simulink model "hexacop"  (R2017a)
settings: Solver=VariableStepAuto  StartTime=0.0  StopTime=10.0  RelTol=1e-3
values from neighbouring files (symbols this model uses):
  b = 3.13*exp(-5)    [Hexacopter_values.m]    (also in values.m)
  d = 7.5*exp(-7)    [values.m]
  g = 9.81    [values.m]
  Jr = 6*exp(-5)    [Hexacopter_values.m]    (also in values.m)
  Jxx = 7.5*10^-3    (= 0.0075)    [Hexacopter_values.m]    (also in values.m = 7.5*exp(-3))
  Jyy = 7.5*10^-3    (= 0.0075)    [Hexacopter_values.m]    (also in values.m = 7.5*exp(-3))
  Jzz = 1.3*10^-2    (= 0.013)    [Hexacopter_values.m]    (also in values.m = 1.3*exp(-2))
  Kfax = 0.1    [Hexacopter_values.m]    (also in values.m)
  Kfay = 0.1    [Hexacopter_values.m]    (also in values.m)
  Kfaz = 0.15    [Hexacopter_values.m]    (also in values.m)
  kftx = 1.5    [values.m]
  kfty = 0.1    [values.m]
  kftz = 1.9    [values.m]
  l = 0.23    [Hexacopter_values.m]    (also in values.m = 1)
  m = 0.65    [Hexacopter_values.m]    (also in values.m = 5)
libraries: simulink x4
settings Model: Creator=Pari  LastModifiedBy=Jash

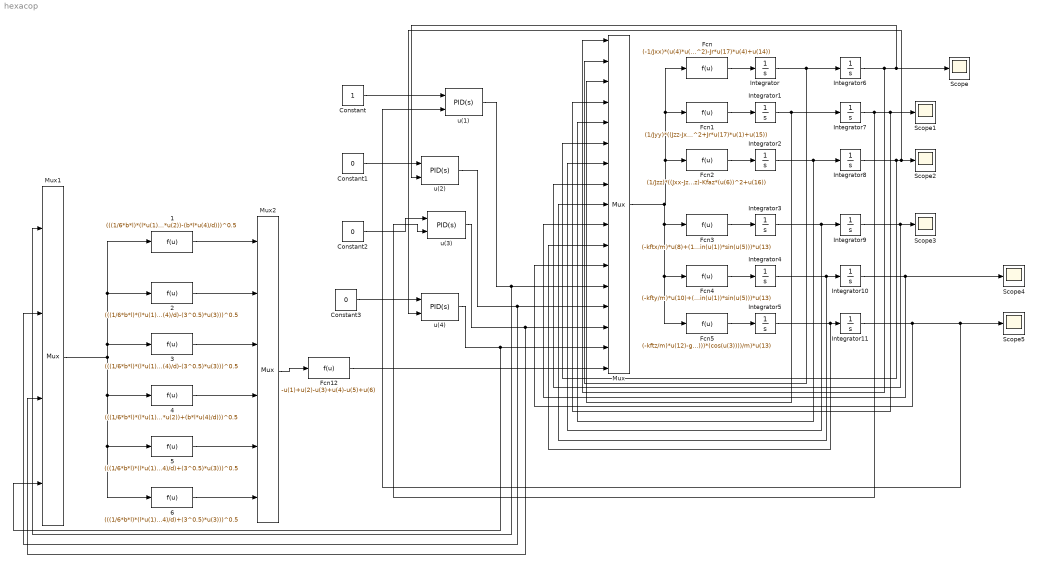
== system hexacop ==
  1 : Fcn  Expr=(((1/6*b*l)*(l*u(1)+2*u(2))-(b*l*u(4)/d)))^0.5
  2 : Fcn  Expr=(((1/6*b*l)*(l*u(1)+u(2))+(b*l*u(4)/d)-(3^0.5)*u(3)))^0.5
  3 : Fcn  Expr=(((1/6*b*l)*(l*u(1)-u(2))-(b*l*u(4)/d)-(3^0.5)*u(3)))^0.5
  4 : Fcn  Expr=(((1/6*b*l)*(l*u(1)-2*u(2))+(b*l*u(4)/d)))^0.5
  5 : Fcn  Expr=(((1/6*b*l)*(l*u(1)-u(2))-(b*l*u(4)/d)+(3^0.5)*u(3)))^0.5
  6 : Fcn  Expr=(((1/6*b*l)*(l*u(1)+u(2))+(b*l*u(4)/d)+(3^0.5)*u(3)))^0.5
  Constant : Constant
  Constant1 : Constant  Value=0
  Constant2 : Constant  Value=0
  Constant3 : Constant  Value=0
  Fcn : Fcn  Expr=(-1/Jxx)*(u(4)*u(6)*(Jyy-Jzz)*Kfax*((u(2))^2)-Jr*u(17)*u(4)+u(14))
  Fcn1 : Fcn  Expr=(1/Jyy)*((Jzz-Jxx)-Kfay*(u(3))^2+Jr*u(17)*u(1)+u(15))
  Fcn12 : Fcn  Expr=-u(1)+u(2)-u(3)+u(4)-u(5)+u(6)
  Fcn2 : Fcn  Expr=(1/Jzz)*((Jxx-Jzz)-Kfaz*(u(6))^2+u(16))
  Fcn3 : Fcn  Expr=(-kftx/m)*u(8)+(1/m)*((cos(u(1))*cos(u(5))*sin(u(3)))+sin(u(1))*sin(u(5)))*u(13)
  Fcn4 : Fcn  Expr=(-kfty/m)*u(10)+(1/m)*((cos(u(1))*sin(u(3))*sin(u(5)))-sin(u(1))*sin(u(5)))*u(13)
  Fcn5 : Fcn  Expr=(-kftz/m)*u(12)-g+(((cos(u(1)))*(cos(u(3))))/m)*u(13)
  Integrator{,1..11} (12 alike) : Integrator
  Mux : Mux  Inputs=17
  Mux1 : Mux
  Mux2 : Mux  Inputs=6
  Scope{,1..5} (6 alike) : Scope
  u(1) : simulink/Continuous/PID Controller (2DOF)  Controller=PID  TimeDomain=Continuous-time  SampleTime=-1  IntegratorMethod=Forward Euler  FilterMethod=Forward Euler  Form=Parallel  UseFilter=on  ControllerParametersSource=internal  P=26.2943879402193  I=7.16633798011478  D=21.031507768883  N=46.9240700820104  b=0.842025544995177  c=0.00338936172316472  InitialConditionSource=internal  InitialConditionForIntegrator=0  InitialConditionForFilter=0  ExternalReset=none  LimitOutput=off  UpperSaturationLimit=inf  LowerSaturationLimit=-inf  LinearizeAsGain=on  AntiWindupMode=none  Kb=1  TrackingMode=off  Kt=1  PParamMin=[]  PParamMax=[]  IParamMin=[]  IParamMax=[]  DParamMin=[]  DParamMax=[]  NParamMin=[]  NParamMax=[]  bParamMin=[]  bParamMax=[]  cParamMin=[]  cParamMax=[]  KbParamMin=[]  KbParamMax=[]  KtParamMin=[]  KtParamMax=[]  POutMin=[]  POutMax=[]  IOutMin=[]  IOutMax=[]  DOutMin=[]  DOutMax=[]  NOutMin=[]  NOutMax=[]  bOutMin=[]  bOutMax=[]  cOutMin=[]  cOutMax=[]  KbOutMin=[]  KbOutMax=[]  KtOutMin=[]  KtOutMax=[]  IntegratorOutMin=[]  IntegratorOutMax=[]  FilterOutMin=[]  FilterOutMax=[]  SumOutMin=[]  SumOutMax=[]  Sum1OutMin=[]  Sum1OutMax=[]  Sum2OutMin=[]  Sum2OutMax=[]  Sum3OutMin=[]  Sum3OutMax=[]  SumI1OutMin=[]  SumI1OutMax=[]  SumI2OutMin=[]  SumI2OutMax=[]  SumI3OutMin=[]  SumI3OutMax=[]  SumDOutMin=[]  SumDOutMax=[]  SaturationOutMin=[]  SaturationOutMax=[]  IntegratorContinuousStateAttributes=''  IntegratorStateMustResolveToSignalObject=off  IntegratorRTWStateStorageClass=Auto  FilterContinuousStateAttributes=''  FilterStateMustResolveToSignalObject=off  FilterRTWStateStorageClass=Auto  DifferentiatorICPrevScaledInput=0  DifferentiatorOutMin=[]  DifferentiatorOutMax=[]  InitialConditionSetting=State (most efficient)
  u(2) : simulink/Continuous/PID Controller (2DOF)  Controller=PID  TimeDomain=Continuous-time  SampleTime=-1  IntegratorMethod=Forward Euler  FilterMethod=Forward Euler  Form=Parallel  UseFilter=on  ControllerParametersSource=internal  P=1  I=1  D=0  N=100  b=1  c=1  InitialConditionSource=internal  InitialConditionForIntegrator=0  InitialConditionForFilter=0  ExternalReset=none  LimitOutput=off  UpperSaturationLimit=inf  LowerSaturationLimit=-inf  LinearizeAsGain=on  AntiWindupMode=none  Kb=1  TrackingMode=off  Kt=1  PParamMin=[]  PParamMax=[]  IParamMin=[]  IParamMax=[]  DParamMin=[]  DParamMax=[]  NParamMin=[]  NParamMax=[]  bParamMin=[]  bParamMax=[]  cParamMin=[]  cParamMax=[]  KbParamMin=[]  KbParamMax=[]  KtParamMin=[]  KtParamMax=[]  POutMin=[]  POutMax=[]  IOutMin=[]  IOutMax=[]  DOutMin=[]  DOutMax=[]  NOutMin=[]  NOutMax=[]  bOutMin=[]  bOutMax=[]  cOutMin=[]  cOutMax=[]  KbOutMin=[]  KbOutMax=[]  KtOutMin=[]  KtOutMax=[]  IntegratorOutMin=[]  IntegratorOutMax=[]  FilterOutMin=[]  FilterOutMax=[]  SumOutMin=[]  SumOutMax=[]  Sum1OutMin=[]  Sum1OutMax=[]  Sum2OutMin=[]  Sum2OutMax=[]  Sum3OutMin=[]  Sum3OutMax=[]  SumI1OutMin=[]  SumI1OutMax=[]  SumI2OutMin=[]  SumI2OutMax=[]  SumI3OutMin=[]  SumI3OutMax=[]  SumDOutMin=[]  SumDOutMax=[]  SaturationOutMin=[]  SaturationOutMax=[]  IntegratorContinuousStateAttributes=''  IntegratorStateMustResolveToSignalObject=off  IntegratorRTWStateStorageClass=Auto  FilterContinuousStateAttributes=''  FilterStateMustResolveToSignalObject=off  FilterRTWStateStorageClass=Auto  DifferentiatorICPrevScaledInput=0  DifferentiatorOutMin=[]  DifferentiatorOutMax=[]  InitialConditionSetting=State (most efficient)
  u(3) : simulink/Continuous/PID Controller (2DOF)  Controller=PID  TimeDomain=Continuous-time  SampleTime=-1  IntegratorMethod=Forward Euler  FilterMethod=Forward Euler  Form=Parallel  UseFilter=on  ControllerParametersSource=internal  P=1  I=1  D=0  N=100  b=1  c=1  InitialConditionSource=internal  InitialConditionForIntegrator=0  InitialConditionForFilter=0  ExternalReset=none  LimitOutput=off  UpperSaturationLimit=inf  LowerSaturationLimit=-inf  LinearizeAsGain=on  AntiWindupMode=none  Kb=1  TrackingMode=off  Kt=1  PParamMin=[]  PParamMax=[]  IParamMin=[]  IParamMax=[]  DParamMin=[]  DParamMax=[]  NParamMin=[]  NParamMax=[]  bParamMin=[]  bParamMax=[]  cParamMin=[]  cParamMax=[]  KbParamMin=[]  KbParamMax=[]  KtParamMin=[]  KtParamMax=[]  POutMin=[]  POutMax=[]  IOutMin=[]  IOutMax=[]  DOutMin=[]  DOutMax=[]  NOutMin=[]  NOutMax=[]  bOutMin=[]  bOutMax=[]  cOutMin=[]  cOutMax=[]  KbOutMin=[]  KbOutMax=[]  KtOutMin=[]  KtOutMax=[]  IntegratorOutMin=[]  IntegratorOutMax=[]  FilterOutMin=[]  FilterOutMax=[]  SumOutMin=[]  SumOutMax=[]  Sum1OutMin=[]  Sum1OutMax=[]  Sum2OutMin=[]  Sum2OutMax=[]  Sum3OutMin=[]  Sum3OutMax=[]  SumI1OutMin=[]  SumI1OutMax=[]  SumI2OutMin=[]  SumI2OutMax=[]  SumI3OutMin=[]  SumI3OutMax=[]  SumDOutMin=[]  SumDOutMax=[]  SaturationOutMin=[]  SaturationOutMax=[]  IntegratorContinuousStateAttributes=''  IntegratorStateMustResolveToSignalObject=off  IntegratorRTWStateStorageClass=Auto  FilterContinuousStateAttributes=''  FilterStateMustResolveToSignalObject=off  FilterRTWStateStorageClass=Auto  DifferentiatorICPrevScaledInput=0  DifferentiatorOutMin=[]  DifferentiatorOutMax=[]  InitialConditionSetting=State (most efficient)
  u(4) : simulink/Continuous/PID Controller (2DOF)  Controller=PID  TimeDomain=Continuous-time  SampleTime=-1  IntegratorMethod=Forward Euler  FilterMethod=Forward Euler  Form=Parallel  UseFilter=on  ControllerParametersSource=internal  P=1  I=1  D=0  N=100  b=1  c=1  InitialConditionSource=internal  InitialConditionForIntegrator=0  InitialConditionForFilter=0  ExternalReset=none  LimitOutput=off  UpperSaturationLimit=inf  LowerSaturationLimit=-inf  LinearizeAsGain=on  AntiWindupMode=none  Kb=1  TrackingMode=off  Kt=1  PParamMin=[]  PParamMax=[]  IParamMin=[]  IParamMax=[]  DParamMin=[]  DParamMax=[]  NParamMin=[]  NParamMax=[]  bParamMin=[]  bParamMax=[]  cParamMin=[]  cParamMax=[]  KbParamMin=[]  KbParamMax=[]  KtParamMin=[]  KtParamMax=[]  POutMin=[]  POutMax=[]  IOutMin=[]  IOutMax=[]  DOutMin=[]  DOutMax=[]  NOutMin=[]  NOutMax=[]  bOutMin=[]  bOutMax=[]  cOutMin=[]  cOutMax=[]  KbOutMin=[]  KbOutMax=[]  KtOutMin=[]  KtOutMax=[]  IntegratorOutMin=[]  IntegratorOutMax=[]  FilterOutMin=[]  FilterOutMax=[]  SumOutMin=[]  SumOutMax=[]  Sum1OutMin=[]  Sum1OutMax=[]  Sum2OutMin=[]  Sum2OutMax=[]  Sum3OutMin=[]  Sum3OutMax=[]  SumI1OutMin=[]  SumI1OutMax=[]  SumI2OutMin=[]  SumI2OutMax=[]  SumI3OutMin=[]  SumI3OutMax=[]  SumDOutMin=[]  SumDOutMax=[]  SaturationOutMin=[]  SaturationOutMax=[]  IntegratorContinuousStateAttributes=''  IntegratorStateMustResolveToSignalObject=off  IntegratorRTWStateStorageClass=Auto  FilterContinuousStateAttributes=''  FilterStateMustResolveToSignalObject=off  FilterRTWStateStorageClass=Auto  DifferentiatorICPrevScaledInput=0  DifferentiatorOutMin=[]  DifferentiatorOutMax=[]  InitialConditionSetting=State (most efficient)
  wires:
  Mux/1 -> Fcn3/1, Fcn4/1, Fcn5/1, Fcn2/1, Fcn1/1, Fcn/1
  Fcn/1 -> Integrator/1
  Fcn3/1 -> Integrator3/1
  Fcn2/1 -> Integrator2/1
  Fcn1/1 -> Integrator1/1
  Fcn4/1 -> Integrator4/1
  Fcn5/1 -> Integrator5/1
  Integrator5/1 -> Mux/11, Integrator11/1
  Integrator4/1 -> Mux/9, Integrator10/1
  Integrator3/1 -> Mux/7, Integrator9/1
  Integrator2/1 -> Mux/5, Integrator8/1
  Integrator1/1 -> Mux/3, Integrator7/1
  Integrator/1 -> Mux/2, Integrator6/1
  Integrator7/1 -> u(3)/2, Mux/4, Scope1/1
  Integrator8/1 -> Mux/6, u(4)/2, Scope2/1
  Integrator9/1 -> Mux/8, Scope3/1
  Integrator10/1 -> Mux/10, Scope4/1
  Integrator11/1 -> Mux/12, u(1)/2, Scope5/1
  Integrator6/1 -> Mux/1, u(2)/2, Scope/1
  Constant/1 -> u(1)/1
  Constant1/1 -> u(2)/1
  Constant2/1 -> u(3)/1
  Constant3/1 -> u(4)/1
  u(1)/1 -> Mux1/1, Mux/13
  u(2)/1 -> Mux1/2, Mux/14
  u(3)/1 -> Mux1/3, Mux/15
  u(4)/1 -> Mux1/4, Mux/16
  Mux1/1 -> 6/1, 5/1, 4/1, 2/1, 1/1, 3/1
  1/1 -> Mux2/1
  2/1 -> Mux2/2
  3/1 -> Mux2/3
  5/1 -> Mux2/5
  6/1 -> Mux2/6
  Mux2/1 -> Fcn12/1
  Fcn12/1 -> Mux/17
  4/1 -> Mux2/4
